simulink library "sm_humanoid_walker_lib"  (R2025b)
settings: Solver=VariableStepAuto  StartTime=0.0  StopTime=10.0  RelTol=1e-3
undefined symbols (not defined in the file or in its folder): params, X, Y, Z
libraries: sm_lib x99, nesl_utility x36, $bdroot x7, simulink x1, simulink_extras x1
(part 1 of 3)
settings Model: Creator=The MathWorks, Inc.  LastModifiedBy=jolson
settings SolverCC: AlgebraicLoopSolver=TrustRegion
settings DebuggingCC: UnconnectedInputMsg=warning  UnconnectedOutputMsg=warning  UnconnectedLineMsg=warning
settings ModelReferenceCC: EnableRefExpFcnMdlSchedulingChecks=on
settings RTWCC: GPUComputeCapability=3.5  DLArmComputeVersion=19.05

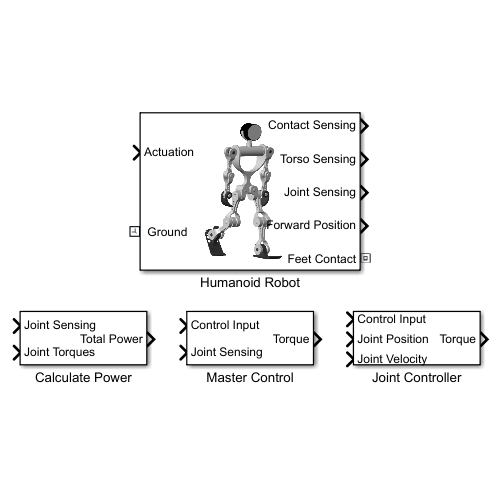
[thumbnail: Simulink's stored preview of the top-level diagram]
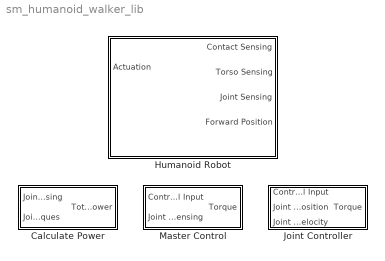
== system sm_humanoid_walker_lib ==
  Calculate Power : Subsystem
  Humanoid Robot : Subsystem  mask{contactRadius=params.contact.contactRadius, contactStiffness=params.contact.stiffness, contactDamping=params.contact.damping, contactTWidth=params.contact.transitionWidth, contactStaticFriction=params.contact.staticFriction, contactDynamicFriction=params.contact.dynamicFriction, contactCriticalVelocity=params.contact.criticalVelocity, footDensity=params.materialProperties.lowerBodyDensity, lowerLegDensity=params.materialProperties.lowerBodyDensity, upperLegDensity=params.materialProperties.lowerBodyDensity, hipDensity=params.materialProperties.lowerBodyDensity, trunkDensity=params.materialProperties.upperBodyDensity, shoulderDensity=params.materialProperties.upperBodyDensity, upperArmDensity=params.materialProperties.upperBodyDensity, lowerArmDensity=params.materialProperties.upperBodyDensity, handDensity=params.materialProperties.upperBodyDensity, headDensity=params.materialProperties.upperBodyDensity, hipUpperLimit=params.jointLimits.hipFrontalUpperLimit, hipLowerLimit=params.jointLimits.hipFrontalLowerLimit, kneeUpperLimit=params.jointLimits.kneeUpperLimit, kneeLowerLimit=params.jointLimits.kneeLowerLimit, ankleUpperLimit=params.jointLimits.ankleUpperLimit, ankleLowerLimit=params.jointLimits.ankleLowerLimit, shoulderFrontalUpperLimit=params.jointLimits.shoulderFrontalUpperLimit, shoulderFrontalLowerLimit=params.jointLimits.shoulderFrontalLowerLimit, shoulderSagittalUpperLimit=params.jointLimits.shoulderSagittalUpperLimit, shoulderSagittalLowerLimit=params.jointLimits.shoulderSagittalLowerLimit}
      mask prompts: contactRadius "Contact Sphere Radius (m)"; contactStiffness "Contact Stiffness (N/m)"; contactDamping "Contact Damping (Ns/m)"; contactTWidth "Contact Tranisiton Region Width (m)"; contactStaticFriction "Contact Static Friction"; contactDynamicFriction "Contact Dynamic Friction"; contactCriticalVelocity "Contact Critical Velocity (m/s)"; footDensity "Foot Density (kg/m^3)"; lowerLegDensity "Lower Leg Density (kg/m^3)"; upperLegDensity "Upper Leg Density (kg/m^3)"; hipDensity "Hip Density (kg/m^3)"; trunkDensity "Trunk Density (kg/m^3)"; shoulderDensity "Shoulder Density (kg/m^3)"; upperArmDensity "Upper Arm Density (kg/m^3)"; lowerArmDensity "Lower Arm Density (kg/m^3)"; handDensity "Hand Density (kg/m^3)"; headDensity "Neck / Head Density (kg/m^3)"; hipUpperLimit "Hip Frontal Upper Limit (deg)"; hipLowerLimit "Hip Frontal Lower Limit (deg)"; kneeUpperLimit "Knee Upper Limit (deg)"; kneeLowerLimit "Knee Lower Limit (deg)"; ankleUpperLimit "Ankle Upper Limit (deg)"; ankleLowerLimit "Ankle Lower Limit (deg)"; shoulderFrontalUpperLimit "Shoulder Frontal Upper Limit (deg)"; shoulderFrontalLowerLimit "Shoulder Frontal Lower Limit (deg)"; shoulderSagittalUpperLimit "Shoulder Sagittal Upper Limit (deg)"; shoulderSagittalLowerLimit "Shoulder Sagittal Lower Limit (deg)"
      mask DialogControl Container4 Prompt: Contact Parameters
      mask DialogControl Container9 Prompt: Material Properties
      mask DialogControl Container12 Prompt: Joint Parameters
      mask Display: image('sm_humanoid_robot.PNG'); % Use "Edit Image" on toolstrip to change.
  Joint Controller : Subsystem  mask{jointStiffness=0, jointDamping=0, jointUpperLimit=0, jointLowerLimit=0, jointTorqueLimit=0}
      mask prompts: jointStiffness "Joint Control Stiffness (N*m/rad)"; jointDamping "Joint Control Damping (N*m*s/rad)"; jointUpperLimit "Joint Upper Limit (deg)"; jointLowerLimit "Joint Lower Limt (deg)"; jointTorqueLimit "Joint Absolute Torque Limit (N*m)"
      mask DialogControl DescTextVar Prompt: Stiffness based joint controller.
  Master Control : Subsystem

== system sm_humanoid_walker_lib/Calculate Power ==
  Joint Sensing : Inport
  Joint Torques : Inport  Port=2
  Bus Selector1 : BusSelector  OutputSignals=signal1.signal1.rhThetaDot,signal1.signal2.rkThetaDot,signal1.signal3.raThetaDot,signal2.signal1.lhThetaDot,signal2.signal2.lkThetaDot,signal2.signal3.laThetaDot
  Mux : Mux  Inputs=6
  Product : Product
  Sum of Elements : Sum  Inputs=+
  Unit Delay : UnitDelay  SampleTime=-1  HasFrameUpgradeWarning=on
  Total Power : Outport
  wires:
  Product/1 -> Sum of Elements/1
  Joint Sensing/1 -> Bus Selector1/1
  Mux/1 -> Product/1
  Joint Torques/1 -> Product/2
  Sum of Elements/1 -> Unit Delay/1
  Bus Selector1/1 -> Mux/1  "<rhThetaDot>"
  Bus Selector1/2 -> Mux/2  "<rkThetaDot>"
  Bus Selector1/3 -> Mux/3  "<raThetaDot>"
  Bus Selector1/4 -> Mux/4  "<lhThetaDot>"
  Bus Selector1/5 -> Mux/5  "<lkThetaDot>"
  Bus Selector1/6 -> Mux/6  "<laThetaDot>"
  Unit Delay/1 -> Total Power/1

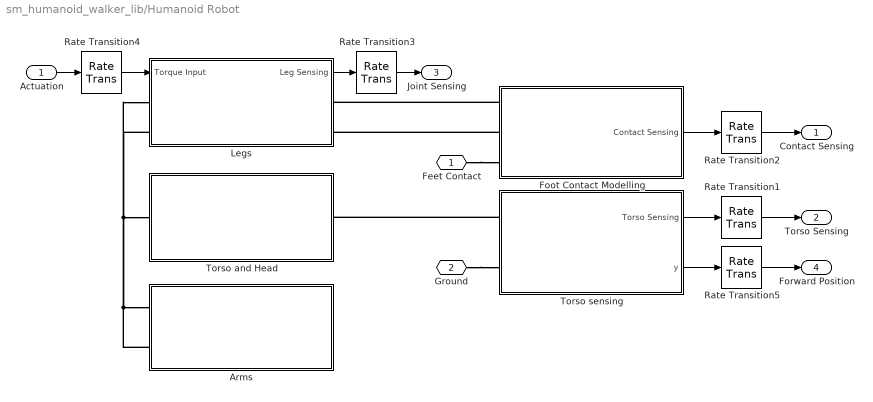
== system sm_humanoid_walker_lib/Humanoid Robot ==
  Actuation : Inport
  Arms : Subsystem
      mask Display: image('sm_humanoid_arms.PNG'); % Use "Edit Image" on toolstrip to change.
  Foot Contact Modelling : Subsystem
  Legs : Subsystem
      mask Display: image('sm_humanoid_legs.PNG'); % Use "Edit Image" on toolstrip to change.
  Rate Transition{1..5} (5 alike) : RateTransition  OutPortSampleTime=params.simulation.Ts
  Torso and Head : Subsystem
      mask Display: image('sm_humanoid_torso.PNG'); % Use "Edit Image" on toolstrip to change.
  Torso sensing : Subsystem
  Feet Contact : PMIOPort  Side=Right
  " Ground" : PMIOPort  Port=2  Side=Left
  Contact Sensing : Outport
  Torso Sensing : Outport  Port=2
  Joint Sensing : Outport  Port=3
  Forward Position : Outport  Port=4
  wires:
  Foot Contact Modelling/1(Contact Sensing) -> Rate Transition2/1
  Legs/1(Leg Sensing) -> Rate Transition3/1
  Actuation/1 -> Rate Transition4/1
  Torso sensing/1(Torso Sensing) -> Rate Transition1/1
  Rate Transition2/1 -> Contact Sensing/1
  Rate Transition1/1 -> Torso Sensing/1
  Rate Transition3/1 -> Joint Sensing/1
  Rate Transition4/1 -> Legs/1(Torque Input)
  Rate Transition5/1 -> Forward Position/1
  Torso sensing/2(y) -> Rate Transition5/1
  connections:
  Arms/LConn2 -- Legs/LConn2 -- Legs/LConn1 -- Torso and Head/LConn1 -- Arms/LConn1
  Torso sensing/LConn1 -- Torso and Head/RConn1
  Feet Contact/RConn1 -- Foot Contact Modelling/LConn3
  Foot Contact Modelling/LConn1 -- Legs/RConn1
  Foot Contact Modelling/LConn2 -- Legs/RConn2
  " Ground"/RConn1 -- Torso sensing/LConn2

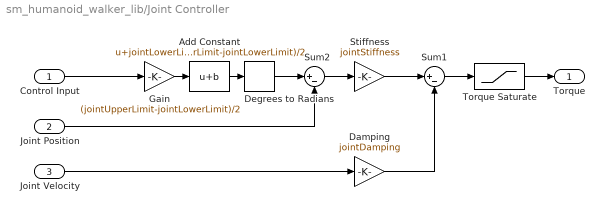
== system sm_humanoid_walker_lib/Joint Controller ==
  Control Input : Inport
  Joint Position : Inport  Port=2
  Joint Velocity : Inport  Port=3
  Add Constant : Bias  Bias=jointLowerLimit + (jointUpperLimit-jointLowerLimit)/2  SaturateOnIntegerOverflow=off
  Damping : Gain  Gain=jointDamping
  Degrees to Radians : simulink_extras/Transformations/Degrees to Radians
  Gain : Gain  Gain=(jointUpperLimit-jointLowerLimit)/2
  Stiffness : Gain  Gain=jointStiffness
  Sum1 : Sum  Inputs=|+-
  Sum2 : Sum  Inputs=|+-
  Torque Saturate : Saturate  UpperLimit=jointTorqueLimit  LowerLimit=-jointTorqueLimit  ZeroCross=off
  Torque : Outport
  wires:
  Damping/1 -> Sum1/2
  Stiffness/1 -> Sum1/1
  Add Constant/1 -> Degrees to Radians/1
  Gain/1 -> Add Constant/1
  Control Input/1 -> Gain/1
  Sum2/1 -> Stiffness/1
  Joint Velocity/1 -> Damping/1
  Sum1/1 -> Torque Saturate/1
  Torque Saturate/1 -> Torque/1
  Degrees to Radians/1 -> Sum2/1
  Joint Position/1 -> Sum2/2

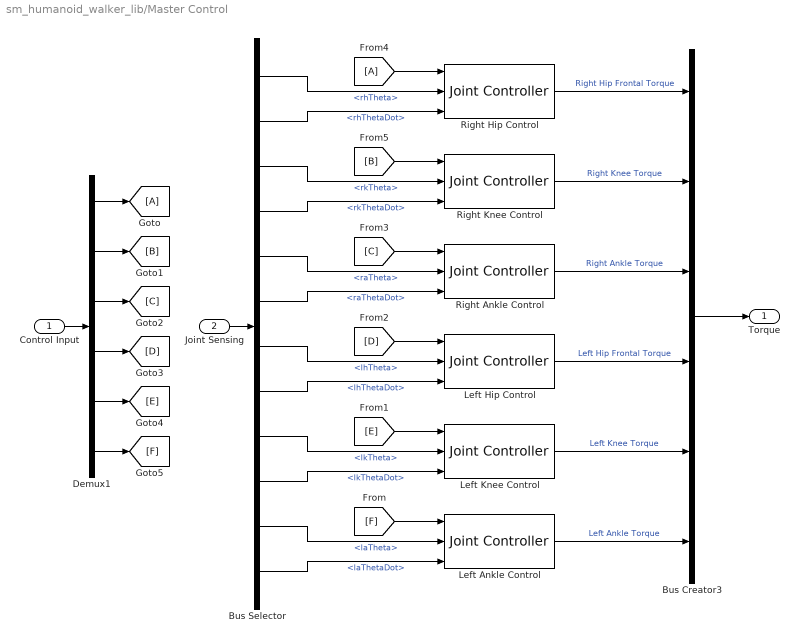
== system sm_humanoid_walker_lib/Master Control ==
  Control Input : Inport
  Joint Sensing : Inport  Port=2
  Bus Creator3 : BusCreator  Inputs=6
  Bus Selector : BusSelector  OutputSignals=signal1.signal1.rhTheta,signal1.signal1.rhThetaDot,signal1.signal2.rkTheta,signal1.signal2.rkThetaDot,signal1.signal3.raTheta,signal1.signal3.raThetaDot,signal2.signal1.lhTheta,signal2.signal1.lhThetaDot,signal2.signal2.lkTheta,signal2.signal2.lkThetaDot,signal2.signal3.laTheta,signal2.signal3.laThetaDot
  Demux1 : Demux  Outputs=6
  From4 : From
  Goto : Goto
  Left Ankle Control : $bdroot/Joint Controller  jointStiffness=params.controller.ankleStiffness  jointDamping=params.controller.ankleDamping  jointUpperLimit=params.jointLimits.ankleUpperLimit  jointLowerLimit=params.jointLimits.ankleLowerLimit  jointTorqueLimit=params.torqueLimits.ankle
  Left Hip Control : $bdroot/Joint Controller  jointStiffness=params.controller.hipFrontalStiffness  jointDamping=params.controller.hipFrontalDamping  jointUpperLimit=params.jointLimits.hipFrontalUpperLimit  jointLowerLimit=params.jointLimits.hipFrontalLowerLimit  jointTorqueLimit=params.torqueLimits.hipFrontal
  Left Knee Control : $bdroot/Joint Controller  jointStiffness=params.controller.kneeStiffness  jointDamping=params.controller.kneeDamping  jointUpperLimit=params.jointLimits.kneeUpperLimit  jointLowerLimit=params.jointLimits.kneeLowerLimit  jointTorqueLimit=params.torqueLimits.knee
  Right Ankle Control : $bdroot/Joint Controller  jointStiffness=params.controller.ankleStiffness  jointDamping=params.controller.ankleDamping  jointUpperLimit=params.jointLimits.ankleUpperLimit  jointLowerLimit=params.jointLimits.ankleLowerLimit  jointTorqueLimit=params.torqueLimits.ankle
  Right Hip Control : $bdroot/Joint Controller  jointStiffness=params.controller.hipFrontalStiffness  jointDamping=params.controller.hipFrontalDamping  jointUpperLimit=params.jointLimits.hipFrontalUpperLimit  jointLowerLimit=params.jointLimits.hipFrontalLowerLimit  jointTorqueLimit=params.torqueLimits.hipFrontal
  Right Knee Control : $bdroot/Joint Controller  jointStiffness=params.controller.kneeStiffness  jointDamping=params.controller.kneeDamping  jointUpperLimit=params.jointLimits.kneeUpperLimit  jointLowerLimit=params.jointLimits.kneeLowerLimit  jointTorqueLimit=params.torqueLimits.knee
  Torque : Outport
  wires:
  Control Input/1 -> Demux1/1
  Joint Sensing/1 -> Bus Selector/1
  Bus Creator3/1 -> Torque/1
  Bus Selector/1 -> Right Hip Control/2  "<rhTheta>"
  Bus Selector/2 -> Right Hip Control/3  "<rhThetaDot>"
  Bus Selector/3 -> Right Knee Control/2  "<rkTheta>"
  Bus Selector/4 -> Right Knee Control/3  "<rkThetaDot>"
  Bus Selector/5 -> Right Ankle Control/2  "<raTheta>"
  Bus Selector/6 -> Right Ankle Control/3  "<raThetaDot>"
  Bus Selector/7 -> Left Hip Control/2  "<lhTheta>"
  Bus Selector/8 -> Left Hip Control/3  "<lhThetaDot>"
  Bus Selector/9 -> Left Knee Control/2  "<lkTheta>"
  Bus Selector/10 -> Left Knee Control/3  "<lkThetaDot>"
  Bus Selector/11 -> Left Ankle Control/2  "<laTheta>"
  Bus Selector/12 -> Left Ankle Control/3  "<laThetaDot>"
  Right Ankle Control/1 -> Bus Creator3/3  "Right Ankle Torque"
  Right Knee Control/1 -> Bus Creator3/2  "Right Knee Torque"
  Right Hip Control/1 -> Bus Creator3/1  "Right Hip Frontal Torque"
  Left Knee Control/1 -> Bus Creator3/5  "Left Knee Torque"
  Left Hip Control/1 -> Bus Creator3/4  "Left Hip Frontal Torque"
  Left Ankle Control/1 -> Bus Creator3/6  "Left Ankle Torque"
  Demux1/1 -> Goto/1
  Demux1/6 -> [F]
  Demux1/5 -> [E]
  Demux1/4 -> [D]
  Demux1/3 -> [C]
  Demux1/2 -> [B]
  [F] -> Left Ankle Control/1
  [E] -> Left Knee Control/1
  [D] -> Left Hip Control/1
  [C] -> Right Ankle Control/1
  From4/1 -> Right Hip Control/1
  [B] -> Right Knee Control/1

== system sm_humanoid_walker_lib/Humanoid Robot/Arms ==
  Left Arm : Subsystem
  Right Arm : Subsystem
  Right Shoulder : PMIOPort  Side=Left
  Left Shoulder : PMIOPort  Port=2  Side=Left
  connections:
  Right Arm/LConn1 -- Right Shoulder/RConn1
  Left Arm/LConn1 -- Left Shoulder/RConn1

== system sm_humanoid_walker_lib/Humanoid Robot/Foot Contact Modelling ==
  Bus Creator : BusCreator  Inputs=2
  Left Foot Contact : $bdroot/Humanoid Robot/Foot Contact Modelling/Right Foot Contact  SystemSampleTime=-1  VariantActivationTime=update diagram  EmptyChoice=off  PassThrough=off  PassThroughVariantControl=(default)  EmptyChoiceVariantControl=(default)  AllowFlexibleInterface=on  Latency=0  AutoFrameSizeCalculation=off
  Right Foot Contact : Subsystem
  Right Foot Contact Points : PMIOPort  Side=Left
  Left Foot Contact Points : PMIOPort  Port=2  Side=Left
  Feet Contact : PMIOPort  Port=3  Side=Left
  Contact Sensing : Outport
  wires:
  Left Foot Contact/1 -> Bus Creator/2  "leftContact"
  Right Foot Contact/1(Foot Force) -> Bus Creator/1  "rightContact"
  Bus Creator/1 -> Contact Sensing/1
  connections:
  Right Foot Contact/LConn1 -- Right Foot Contact Points/RConn1
  Right Foot Contact/RConn1 -- Left Foot Contact/RConn1 -- Feet Contact/RConn1
  Left Foot Contact/LConn1 -- Left Foot Contact Points/RConn1

== system sm_humanoid_walker_lib/Humanoid Robot/Legs ==
  Torque Input : Inport
  Bus Creator1 : BusCreator  Inputs=2
  Demux : Demux  Outputs=2
  Left Leg : Subsystem
  Right leg : Subsystem
  Right Hip : PMIOPort  Side=Left
  Right Foot : PMIOPort  Port=2  Side=Right
  Left Foot : PMIOPort  Port=3  Side=Right
  Left Hip : PMIOPort  Port=4  Side=Left
  Leg Sensing : Outport
  wires:
  Demux/1 -> Right leg/1(Torque Input)
  Torque Input/1 -> Demux/1
  Left Leg/1(Sensing) -> Bus Creator1/2
  Right leg/1(Sensing) -> Bus Creator1/1
  Bus Creator1/1 -> Leg Sensing/1
  Demux/2 -> Left Leg/1(Torque Input)
  connections:
  Left Hip/RConn1 -- Left Leg/LConn1
  Right Foot/RConn1 -- Right leg/RConn1
  Left Foot/RConn1 -- Left Leg/RConn1
  Right Hip/RConn1 -- Right leg/LConn1

== system sm_humanoid_walker_lib/Humanoid Robot/Torso and Head ==
  Cover : sm_lib/Body Elements/File Solid  ExtGeomFileName=sm_humanoid_walker_cover.stp  UnitType=FromFile  ExtGeomFileUnits=m  StepReaderType=HEX  ExportConvexHullGeometry=off  InertiaType=CalculateFromGeometry  BasedOnType=Density  Density=headDensity  DensityUnits=kg/m^3  Mass=0  MassUnits=kg  CenterOfMass=[0, 0, 0]  CenterOfMassUnits=m  MomentsOfInertia=[0, 0, 0]  MomentsOfInertiaUnits=kg*m^2  ProductsOfInertia=[0, 0, 0]  ProductsOfInertiaUnits=kg*m^2  GraphicType=FromGeometry  MarkerShape=Sphere  MarkerSize=10  GraphicVisPropType=SimpleVisualProperties  GraphicDiffuseColor=[1, 1, 1]  GraphicOpacity=1  GraphicSpecularColor=[0.5 0.5 0.5 1.0]  GraphicAmbientColor=[0.15 0.15 0.15 1.0]  GraphicEmissiveColor=[0.0 0.0 0.0 1.0]  GraphicShininess=75  DoExposeReferenceFrame=on  SerializedFrames=<Frames/>
  Head : sm_lib/Body Elements/File Solid  ExtGeomFileName=sm_humanoid_walker_head.stp  UnitType=FromFile  ExtGeomFileUnits=m  StepReaderType=HEX  ExportConvexHullGeometry=off  InertiaType=CalculateFromGeometry  BasedOnType=Density  Density=headDensity  DensityUnits=kg/m^3  Mass=0  MassUnits=kg  CenterOfMass=[0, 0, 0]  CenterOfMassUnits=m  MomentsOfInertia=[0, 0, 0]  MomentsOfInertiaUnits=kg*m^2  ProductsOfInertia=[0, 0, 0]  ProductsOfInertiaUnits=kg*m^2  GraphicType=FromGeometry  MarkerShape=Sphere  MarkerSize=10  GraphicVisPropType=SimpleVisualProperties  GraphicDiffuseColor=[0.0 0.0 0.0]  GraphicOpacity=1  GraphicSpecularColor=[0.5 0.5 0.5 1.0]  GraphicAmbientColor=[0.15 0.15 0.15 1.0]  GraphicEmissiveColor=[0.0 0.0 0.0 1.0]  GraphicShininess=75  DoExposeReferenceFrame=on  SerializedFrames=<Frames/>
  Head Origin Transformation : sm_lib/Frames and Transforms/Rigid Transform  RotationMethod=RotationSequence  FollAlignAxisA=+X  BaseAlignAxisA=+Y  FollAlignAxisB=+Y  BaseAlignAxisB=+Z  RotationStandardAxis=+Z  RotationAngle=0.0  RotationAngleUnits=deg  RotationArbitraryAxis=[0 0 1]  RotationSequenceAxes=BaseAxes  RotationSequence=XYZ  RotationSequenceAngles=[0, 0, 0]  RotationSequenceAnglesUnits=rad  RotationMatrix=[1 0 0; 0 1 0; 0 0 1]  Quaternion=[1 0 0 0]  TranslationMethod=Cartesian  TranslationCartesianOffset=[0, 0, 0.06414]*3.5  TranslationCartesianOffsetUnits=m  TranslationStandardAxis=+Z  TranslationStandardOffset=0  TranslationStandardOffsetUnits=m  TranslationROffset=0  TranslationROffsetUnits=m  TranslationThetaOffset=0  TranslationThetaOffsetUnits=deg  TranslationZOffset=0  TranslationZOffsetUnits=m
  Neck : sm_lib/Body Elements/File Solid  ExtGeomFileName=sm_humanoid_walker_neck.stp  UnitType=FromFile  ExtGeomFileUnits=m  StepReaderType=HEX  ExportConvexHullGeometry=off  InertiaType=CalculateFromGeometry  BasedOnType=Density  Density=headDensity  DensityUnits=kg/m^3  Mass=0  MassUnits=kg  CenterOfMass=[0, 0, 0]  CenterOfMassUnits=m  MomentsOfInertia=[0, 0, 0]  MomentsOfInertiaUnits=kg*m^2  ProductsOfInertia=[0, 0, 0]  ProductsOfInertiaUnits=kg*m^2  GraphicType=FromGeometry  MarkerShape=Sphere  MarkerSize=10  GraphicVisPropType=SimpleVisualProperties  GraphicDiffuseColor=[0.0 0.0 0.0]  GraphicOpacity=1  GraphicSpecularColor=[0.5 0.5 0.5 1.0]  GraphicAmbientColor=[0.15 0.15 0.15 1.0]  GraphicEmissiveColor=[0.0 0.0 0.0 1.0]  GraphicShininess=75  DoExposeReferenceFrame=on  SerializedFrames=<Frames/>
  Neck Origin Tranformation : sm_lib/Frames and Transforms/Rigid Transform  RotationMethod=RotationSequence  FollAlignAxisA=+X  BaseAlignAxisA=+Y  FollAlignAxisB=+Y  BaseAlignAxisB=+Z  RotationStandardAxis=+Z  RotationAngle=0.0  RotationAngleUnits=deg  RotationArbitraryAxis=[0 0 1]  RotationSequenceAxes=BaseAxes  RotationSequence=XYZ  RotationSequenceAngles=[0, 0, 0]  RotationSequenceAnglesUnits=rad  RotationMatrix=[1 0 0; 0 1 0; 0 0 1]  Quaternion=[1 0 0 0]  TranslationMethod=Cartesian  TranslationCartesianOffset=[0, 0, 0.01016]*3.5  TranslationCartesianOffsetUnits=m  TranslationStandardAxis=+Z  TranslationStandardOffset=0  TranslationStandardOffsetUnits=m  TranslationROffset=0  TranslationROffsetUnits=m  TranslationThetaOffset=0  TranslationThetaOffsetUnits=deg  TranslationZOffset=0  TranslationZOffsetUnits=m
  Shoulder : sm_lib/Body Elements/File Solid  ExtGeomFileName=sm_humanoid_walker_shoulder.stp  UnitType=FromFile  ExtGeomFileUnits=m  StepReaderType=HEX  ExportConvexHullGeometry=off  InertiaType=CalculateFromGeometry  BasedOnType=Density  Density=shoulderDensity  DensityUnits=kg/m^3  Mass=0  MassUnits=kg  CenterOfMass=[0, 0, 0]  CenterOfMassUnits=m  MomentsOfInertia=[0, 0, 0]  MomentsOfInertiaUnits=kg*m^2  ProductsOfInertia=[0, 0, 0]  ProductsOfInertiaUnits=kg*m^2  GraphicType=FromGeometry  MarkerShape=Sphere  MarkerSize=10  GraphicVisPropType=SimpleVisualProperties  GraphicDiffuseColor=[1.0 0.6 0.6]  GraphicOpacity=1  GraphicSpecularColor=[0.5 0.5 0.5 1.0]  GraphicAmbientColor=[0.15 0.15 0.15 1.0]  GraphicEmissiveColor=[0.0 0.0 0.0 1.0]  GraphicShininess=75  DoExposeReferenceFrame=on  SerializedFrames=<Frames/>
  Shoulder Origin Transformation : sm_lib/Frames and Transforms/Rigid Transform  RotationMethod=RotationSequence  FollAlignAxisA=+X  BaseAlignAxisA=+Y  FollAlignAxisB=+Y  BaseAlignAxisB=+Z  RotationStandardAxis=+Z  RotationAngle=0.0  RotationAngleUnits=deg  RotationArbitraryAxis=[0 0 1]  RotationSequenceAxes=BaseAxes  RotationSequence=XYZ  RotationSequenceAngles=[0, 0, 0]  RotationSequenceAnglesUnits=rad  RotationMatrix=[1 0 0; 0 1 0; 0 0 1]  Quaternion=[1 0 0 0]  TranslationMethod=Cartesian  TranslationCartesianOffset=[0, 0, -0.0399]*3.5  TranslationCartesianOffsetUnits=m  TranslationStandardAxis=+Z  TranslationStandardOffset=0  TranslationStandardOffsetUnits=m  TranslationROffset=0  TranslationROffsetUnits=m  TranslationThetaOffset=0  TranslationThetaOffsetUnits=deg  TranslationZOffset=0  TranslationZOffsetUnits=m
  Trunk : sm_lib/Body Elements/File Solid  ExtGeomFileName=sm_humanoid_walker_trunk.stp  UnitType=FromFile  ExtGeomFileUnits=km  StepReaderType=HEX  ExportConvexHullGeometry=off  InertiaType=CalculateFromGeometry  BasedOnType=Density  Density=trunkDensity  DensityUnits=kg/m^3  Mass=0  MassUnits=kg  CenterOfMass=[0, 0, 0]  CenterOfMassUnits=m  MomentsOfInertia=[0, 0, 0]  MomentsOfInertiaUnits=kg*m^2  ProductsOfInertia=[0, 0, 0]  ProductsOfInertiaUnits=kg*m^2  GraphicType=FromGeometry  MarkerShape=Sphere  MarkerSize=10  GraphicVisPropType=SimpleVisualProperties  GraphicDiffuseColor=[1.0 0.2 0.2]  GraphicOpacity=1  GraphicSpecularColor=[0.5 0.5 0.5 1.0]  GraphicAmbientColor=[0.15 0.15 0.15 1.0]  GraphicEmissiveColor=[0.0 0.0 0.0 1.0]  GraphicShininess=75  DoExposeReferenceFrame=on  SerializedFrames=<Frames/>
  Torso : PMIOPort  Side=Left
  Torso Ref : PMIOPort  Port=2  Side=Right
  connections:
  Shoulder Origin Transformation/LConn1 -- Torso Ref/RConn1 -- Torso/RConn1 -- Trunk/RConn1
  Head/RConn1 -- Head Origin Transformation/RConn1 -- Cover/RConn1
  Shoulder/RConn1 -- Shoulder Origin Transformation/RConn1 -- Neck Origin Tranformation/LConn1
  Neck Origin Tranformation/RConn1 -- Head Origin Transformation/LConn1 -- Neck/RConn1

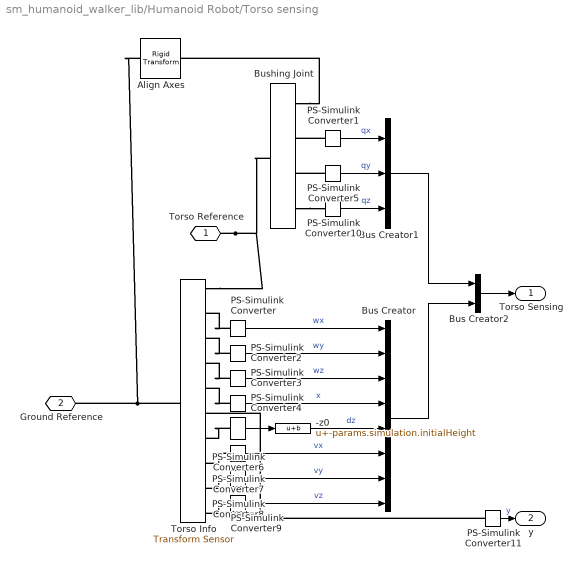
== system sm_humanoid_walker_lib/Humanoid Robot/Torso sensing ==
  -z0 : Bias  Bias=-params.simulation.initialHeight  SaturateOnIntegerOverflow=off
  Align Axes : sm_lib/Frames and Transforms/Rigid Transform  RotationMethod=StandardAxis  FollAlignAxisA=+X  BaseAlignAxisA=+Y  FollAlignAxisB=+Y  BaseAlignAxisB=+Z  RotationStandardAxis=+Z  RotationAngle=180  RotationAngleUnits=deg  RotationArbitraryAxis=[0 0 1]  RotationSequenceAxes=FollowerAxes  RotationSequence=XYX  RotationSequenceAngles=[0 0 0]  RotationSequenceAnglesUnits=deg  RotationMatrix=[1 0 0; 0 1 0; 0 0 1]  Quaternion=[1 0 0 0]  TranslationMethod=None  TranslationCartesianOffset=[0 0 0]  TranslationCartesianOffsetUnits=m  TranslationStandardAxis=+Z  TranslationStandardOffset=0  TranslationStandardOffsetUnits=m  TranslationROffset=0  TranslationROffsetUnits=m  TranslationThetaOffset=0  TranslationThetaOffsetUnits=deg  TranslationZOffset=0  TranslationZOffsetUnits=m
  Bus Creator : BusCreator  Inputs=8
  Bus Creator1 : BusCreator  Inputs=3
  Bus Creator2 : BusCreator  Inputs=2
  Bushing Joint : sm_lib/Joints/Bushing Joint  JointMode=Normal  CompositeWrenchDir=FollowerOnBase  CompositeWrenchFrame=BaseFrame  SenseConstraintForce=off  SenseConstraintTorque=off  SenseTotalForce=off  SenseTotalTorque=off  PxPositionTargetSpecify=off  PxPositionTargetPriority=High  PxPositionTargetValue=0  PxPositionTargetValueUnits=m  PxVelocityTargetSpecify=off  PxVelocityTargetPriority=High  PxVelocityTargetValue=0  PxVelocityTargetValueUnits=m/s  PxEquilibriumPosition=0  PxEquilibriumPositionUnits=m  PxSpringStiffness=0  PxSpringStiffnessUnits=N/m  PxDampingCoefficient=0  PxDampingCoefficientUnits=N/(m/s)  PxLowerLimitSpecify=off  PxLowerLimitBound=-0.02  PxLowerLimitBoundUnits=m  PxLowerLimitStiffness=1e6  PxLowerLimitStiffnessUnits=N/m  PxLowerLimitDamping=1e3  PxLowerLimitDampingUnits=N/(m/s)  PxLowerLimitTransitionRegionWidth=1e-4  PxLowerLimitTransitionRegionWidthUnits=m  PxUpperLimitSpecify=off  PxUpperLimitBound=0.02  PxUpperLimitBoundUnits=m  PxUpperLimitStiffness=1e6  PxUpperLimitStiffnessUnits=N/m  PxUpperLimitDamping=1e3  PxUpperLimitDampingUnits=N/(m/s)  PxUpperLimitTransitionRegionWidth=1e-4  PxUpperLimitTransitionRegionWidthUnits=m  PxTorqueActuationMode=NoTorque  PxMotionActuationMode=ComputedMotion  PxSensePosition=off  PxSenseVelocity=off  PxSenseAcceleration=off  PxSenseTorqueForce=off  PxSenseLowerLimitTorqueForce=off  PxSenseUpperLimitTorqueForce=off  PyPositionTargetSpecify=off  PyPositionTargetPriority=High  PyPositionTargetValue=0  PyPositionTargetValueUnits=m  PyVelocityTargetSpecify=off  PyVelocityTargetPriority=High  PyVelocityTargetValue=0  PyVelocityTargetValueUnits=m/s  PyEquilibriumPosition=0  PyEquilibriumPositionUnits=m  PySpringStiffness=0  PySpringStiffnessUnits=N/m  PyDampingCoefficient=0  PyDampingCoefficientUnits=N/(m/s)  PyLowerLimitSpecify=off  PyLowerLimitBound=-1  PyLowerLimitBoundUnits=m  PyLowerLimitStiffness=1e6  PyLowerLimitStiffnessUnits=N/m  PyLowerLimitDamping=1e3  PyLowerLimitDampingUnits=N/(m/s)  PyLowerLimitTransitionRegionWidth=1e-4  PyLowerLimitTransitionRegionWidthUnits=m  PyUpperLimitSpecify=off  PyUpperLimitBound=1  PyUpperLimitBoundUnits=m  PyUpperLimitStiffness=1e6  PyUpperLimitStiffnessUnits=N/m  PyUpperLimitDamping=1e3  PyUpperLimitDampingUnits=N/(m/s)  PyUpperLimitTransitionRegionWidth=1e-4  PyUpperLimitTransitionRegionWidthUnits=m  PyTorqueActuationMode=NoTorque  PyMotionActuationMode=ComputedMotion  PySensePosition=off  PySenseVelocity=off  PySenseAcceleration=off  PySenseTorqueForce=off  PySenseLowerLimitTorqueForce=off  PySenseUpperLimitTorqueForce=off  PzPositionTargetSpecify=on  PzPositionTargetPriority=High  PzPositionTargetValue=-params.simulation.initialHeight  PzPositionTargetValueUnits=m  PzVelocityTargetSpecify=off  PzVelocityTargetPriority=High  PzVelocityTargetValue=0  PzVelocityTargetValueUnits=m/s  PzEquilibriumPosition=0  PzEquilibriumPositionUnits=m  PzSpringStiffness=0  PzSpringStiffnessUnits=N/m  PzDampingCoefficient=params.simulation.worldDamping  PzDampingCoefficientUnits=N/(m/s)  PzLowerLimitSpecify=off  PzLowerLimitBound=-1  PzLowerLimitBoundUnits=m  PzLowerLimitStiffness=1e6  PzLowerLimitStiffnessUnits=N/m  PzLowerLimitDamping=1e3  PzLowerLimitDampingUnits=N/(m/s)  PzLowerLimitTransitionRegionWidth=1e-4  PzLowerLimitTransitionRegionWidthUnits=m  PzUpperLimitSpecify=off  PzUpperLimitBound=1  PzUpperLimitBoundUnits=m  PzUpperLimitStiffness=1e6  PzUpperLimitStiffnessUnits=N/m  PzUpperLimitDamping=1e3  PzUpperLimitDampingUnits=N/(m/s)  PzUpperLimitTransitionRegionWidth=1e-4  PzUpperLimitTransitionRegionWidthUnits=m  PzTorqueActuationMode=NoTorque  PzMotionActuationMode=ComputedMotion  PzSensePosition=off  PzSenseVelocity=off  PzSenseAcceleration=off  PzSenseTorqueForce=off  PzSenseLowerLimitTorqueForce=off  PzSenseUpperLimitTorqueForce=off  RxPositionTargetSpecify=on  RxPositionTargetPriority=High  RxPositionTargetValue=-10  RxPositionTargetValueUnits=deg  RxVelocityTargetSpecify=off  RxVelocityTargetPriority=High  RxVelocityTargetValue=0  RxVelocityTargetValueUnits=deg/s  RxEquilibriumPosition=0  RxEquilibriumPositionUnits=deg  RxSpringStiffness=0  RxSpringStiffnessUnits=N*m/deg  RxDampingCoefficient=params.simulation.worldDamping  RxDampingCoefficientUnits=N*m/(deg/s)  RxLowerLimitSpecify=off  RxLowerLimitBound=-90  RxLowerLimitBoundUnits=deg  RxLowerLimitStiffness=1e4  RxLowerLimitStiffnessUnits=N*m/deg  RxLowerLimitDamping=10  RxLowerLimitDampingUnits=N*m/(deg/s)  RxLowerLimitTransitionRegionWidth=0.1  RxLowerLimitTransitionRegionWidthUnits=deg  RxUpperLimitSpecify=off  RxUpperLimitBound=90  RxUpperLimitBoundUnits=deg  RxUpperLimitStiffness=1e4  RxUpperLimitStiffnessUnits=N*m/deg  RxUpperLimitDamping=10  RxUpperLimitDampingUnits=N*m/(deg/s)  RxUpperLimitTransitionRegionWidth=0.1  RxUpperLimitTransitionRegionWidthUnits=deg  RxTorqueActuationMode=NoTorque  RxMotionActuationMode=ComputedMotion  RxSensePosition=on  RxSenseVelocity=off  RxSenseAcceleration=off  RxSenseTorqueForce=off  RxSenseLowerLimitTorqueForce=off  RxSenseUpperLimitTorqueForce=off  RyPositionTargetSpecify=off  RyPositionTargetPriority=High  RyPositionTargetValue=0  RyPositionTargetValueUnits=deg  RyVelocityTargetSpecify=off  RyVelocityTargetPriority=High  RyVelocityTargetValue=0  RyVelocityTargetValueUnits=deg/s  RyEquilibriumPosition=0  RyEquilibriumPositionUnits=deg  RySpringStiffness=0  RySpringStiffnessUnits=N*m/deg  RyDampingCoefficient=params.simulation.worldDamping  RyDampingCoefficientUnits=N*m/(deg/s)  RyLowerLimitSpecify=off  RyLowerLimitBound=-90  RyLowerLimitBoundUnits=deg  RyLowerLimitStiffness=1e4  RyLowerLimitStiffnessUnits=N*m/deg  RyLowerLimitDamping=10  RyLowerLimitDampingUnits=N*m/(deg/s)  RyLowerLimitTransitionRegionWidth=0.1  RyLowerLimitTransitionRegionWidthUnits=deg  RyUpperLimitSpecify=off  RyUpperLimitBound=90  RyUpperLimitBoundUnits=deg  RyUpperLimitStiffness=1e4  RyUpperLimitStiffnessUnits=N*m/deg  RyUpperLimitDamping=10  RyUpperLimitDampingUnits=N*m/(deg/s)  RyUpperLimitTransitionRegionWidth=0.1  RyUpperLimitTransitionRegionWidthUnits=deg  RyTorqueActuationMode=NoTorque  RyMotionActuationMode=ComputedMotion  RySensePosition=on  RySenseVelocity=off  RySenseAcceleration=off  RySenseTorqueForce=off  RySenseLowerLimitTorqueForce=off  RySenseUpperLimitTorqueForce=off  RzPositionTargetSpecify=on  RzPositionTargetPriority=High  RzPositionTargetValue=0  RzPositionTargetValueUnits=deg  RzVelocityTargetSpecify=off  RzVelocityTargetPriority=High  RzVelocityTargetValue=0  RzVelocityTargetValueUnits=deg/s  RzEquilibriumPosition=0  RzEquilibriumPositionUnits=deg  RzSpringStiffness=0  RzSpringStiffnessUnits=N*m/deg  RzDampingCoefficient=params.simulation.worldDamping  RzDampingCoefficientUnits=N*m/(deg/s)  RzLowerLimitSpecify=off  RzLowerLimitBound=-90  RzLowerLimitBoundUnits=deg  RzLowerLimitStiffness=1e4  RzLowerLimitStiffnessUnits=N*m/deg  RzLowerLimitDamping=10  RzLowerLimitDampingUnits=N*m/(deg/s)  RzLowerLimitTransitionRegionWidth=0.1  RzLowerLimitTransitionRegionWidthUnits=deg  RzUpperLimitSpecify=off  RzUpperLimitBound=90  RzUpperLimitBoundUnits=deg  RzUpperLimitStiffness=1e4  RzUpperLimitStiffnessUnits=N*m/deg  RzUpperLimitDamping=10  RzUpperLimitDampingUnits=N*m/(deg/s)  RzUpperLimitTransitionRegionWidth=0.1  RzUpperLimitTransitionRegionWidthUnits=deg  RzTorqueActuationMode=NoTorque  RzMotionActuationMode=ComputedMotion  RzSensePosition=on  RzSenseVelocity=off  RzSenseAcceleration=off  RzSenseTorqueForce=off  RzSenseLowerLimitTorqueForce=off  RzSenseUpperLimitTorqueForce=off
  PS-Simulink Converter{,1..11} (12 alike) : nesl_utility/PS-Simulink Converter  PhysicalDomain=network_engine_domain  SubClassName=ps_output  LeftPortType=input  RightPortType=output  PseudoPeriodic=off  Frequencies=[]  VectorFormat=1-D array  Unit=inherit  AffineConversion=off
  Torso Info : sm_lib/Frames and Transforms/Transform Sensor  MeasurementFrame=World  RotationSequence=XYX  SenseAngle=off  SenseAxis=off  SenseQ=off  SenseR=off  SenseRotationSequence=off  SenseOmegaX=on  SenseOmegaY=on  SenseOmegaZ=on  SenseOmega=off  SenseQDot=off  SenseRDot=off  SenseRotationSequenceDot=off  SenseAlphaX=off  SenseAlphaY=off  SenseAlphaZ=off  SenseAlpha=off  SenseQDDot=off  SenseRDDot=off  SenseX=on  SenseY=on  SenseZ=on  SenseXYZ=off  SenseRad=off  SenseAzim=off  SenseDist=off  SenseInc=off  SenseXDot=on  SenseYDot=on  SenseZDot=on  SenseXYZDot=off  SenseRadDot=off  SenseAzimDot=off  SenseDistDot=off  SenseIncDot=off  SenseXDDot=off  SenseYDDot=off  SenseZDDot=off  SenseXYZDDot=off  SenseRadDDot=off  SenseAzimDDot=off  SenseDistDDot=off  SenseIncDDot=off
  Torso Reference : PMIOPort  Side=Left
  Ground Reference : PMIOPort  Port=2  Side=Left
  Torso Sensing : Outport
  y : Outport  Port=2
  wires:
  Bus Creator/1 -> Bus Creator2/2
  Bus Creator2/1 -> Torso Sensing/1
  PS-Simulink Converter1/1 -> Bus Creator1/1  "qx"
  PS-Simulink Converter5/1 -> Bus Creator1/2  "qy"
  Bus Creator1/1 -> Bus Creator2/1
  PS-Simulink Converter10/1 -> Bus Creator1/3  "qz"
  -z0/1 -> Bus Creator/5  "dz"
  PS-Simulink Converter9/1 -> Bus Creator/8  "vz"
  PS-Simulink Converter8/1 -> Bus Creator/7  "vy"
  PS-Simulink Converter7/1 -> Bus Creator/6  "vx"
  PS-Simulink Converter6/1 -> -z0/1
  PS-Simulink Converter4/1 -> Bus Creator/4  "x"
  PS-Simulink Converter3/1 -> Bus Creator/3  "wz"
  PS-Simulink Converter2/1 -> Bus Creator/2  "wy"
  PS-Simulink Converter/1 -> Bus Creator/1  "wx"
  PS-Simulink Converter11/1 -> y/1  "y"
  connections:
  Torso Info/LConn1 -- Ground Reference/RConn1 -- Align Axes/LConn1
  PS-Simulink Converter1/LConn1 -- Bushing Joint/RConn2
  PS-Simulink Converter5/LConn1 -- Bushing Joint/RConn3
  Bushing Joint/RConn4 -- PS-Simulink Converter10/LConn1
  PS-Simulink Converter2/LConn1 -- Torso Info/RConn3
  PS-Simulink Converter3/LConn1 -- Torso Info/RConn4
  PS-Simulink Converter4/LConn1 -- Torso Info/RConn5
  PS-Simulink Converter/LConn1 -- Torso Info/RConn2
  Bushing Joint/RConn1 -- Align Axes/RConn1
  Torso Reference/RConn1 -- Bushing Joint/LConn1 -- Torso Info/RConn1
  PS-Simulink Converter9/LConn1 -- Torso Info/RConn10
  PS-Simulink Converter8/LConn1 -- Torso Info/RConn9
  PS-Simulink Converter7/LConn1 -- Torso Info/RConn8
  PS-Simulink Converter6/LConn1 -- Torso Info/RConn7
  PS-Simulink Converter11/LConn1 -- Torso Info/RConn6

== system sm_humanoid_walker_lib/Humanoid Robot/Arms/Left Arm ==
  Elbow Joint : Subsystem
  Hand : sm_lib/Body Elements/File Solid  ExtGeomFileName=sm_humanoid_walker_hand.stp  UnitType=FromFile  ExtGeomFileUnits=m  StepReaderType=HEX  ExportConvexHullGeometry=off  InertiaType=CalculateFromGeometry  BasedOnType=Density  Density=handDensity  DensityUnits=kg/m^3  Mass=0  MassUnits=kg  CenterOfMass=[0, 0, 0]  CenterOfMassUnits=m  MomentsOfInertia=[0, 0, 0]  MomentsOfInertiaUnits=kg*m^2  ProductsOfInertia=[0, 0, 0]  ProductsOfInertiaUnits=kg*m^2  GraphicType=FromGeometry  MarkerShape=Sphere  MarkerSize=10  GraphicVisPropType=SimpleVisualProperties  GraphicDiffuseColor=[0.3, 0.3, 0.3]  GraphicOpacity=1  GraphicSpecularColor=[0.5 0.5 0.5 1.0]  GraphicAmbientColor=[0.15 0.15 0.15 1.0]  GraphicEmissiveColor=[0.0 0.0 0.0 1.0]  GraphicShininess=75  DoExposeReferenceFrame=on  SerializedFrames=<Frames/>
  Lower Arm : sm_lib/Body Elements/File Solid  ExtGeomFileName=sm_humanoid_walker_lower_arm.stp  UnitType=FromFile  ExtGeomFileUnits=m  StepReaderType=HEX  ExportConvexHullGeometry=off  InertiaType=CalculateFromGeometry  BasedOnType=Density  Density=lowerArmDensity  DensityUnits=kg/m^3  Mass=0  MassUnits=kg  CenterOfMass=[0, 0, 0]  CenterOfMassUnits=m  MomentsOfInertia=[0, 0, 0]  MomentsOfInertiaUnits=kg*m^2  ProductsOfInertia=[0, 0, 0]  ProductsOfInertiaUnits=kg*m^2  GraphicType=FromGeometry  MarkerShape=Sphere  MarkerSize=10  GraphicVisPropType=SimpleVisualProperties  GraphicDiffuseColor=[1, 1, 1]  GraphicOpacity=1  GraphicSpecularColor=[0.5 0.5 0.5 1.0]  GraphicAmbientColor=[0.15 0.15 0.15 1.0]  GraphicEmissiveColor=[0.0 0.0 0.0 1.0]  GraphicShininess=75  DoExposeReferenceFrame=on  SerializedFrames=<Frames/>
  Shoulder Frontal Joint : Subsystem
  Shoulder Sagittal Joint : Subsystem
  Shoulder Swivel : sm_lib/Body Elements/File Solid  ExtGeomFileName=sm_humanoid_walker_shoulder_swivel.stp  UnitType=FromFile  ExtGeomFileUnits=m  StepReaderType=HEX  ExportConvexHullGeometry=off  InertiaType=CalculateFromGeometry  BasedOnType=Density  Density=shoulderDensity  DensityUnits=kg/m^3  Mass=0  MassUnits=kg  CenterOfMass=[0, 0, 0]  CenterOfMassUnits=m  MomentsOfInertia=[0, 0, 0]  MomentsOfInertiaUnits=kg*m^2  ProductsOfInertia=[0, 0, 0]  ProductsOfInertiaUnits=kg*m^2  GraphicType=FromGeometry  MarkerShape=Sphere  MarkerSize=10  GraphicVisPropType=SimpleVisualProperties  GraphicDiffuseColor=[0.3, 0.3, 0.3]  GraphicOpacity=1  GraphicSpecularColor=[0.5 0.5 0.5 1.0]  GraphicAmbientColor=[0.15 0.15 0.15 1.0]  GraphicEmissiveColor=[0.0 0.0 0.0 1.0]  GraphicShininess=75  DoExposeReferenceFrame=on  SerializedFrames=<Frames/>
  Upper Arm : sm_lib/Body Elements/File Solid  ExtGeomFileName=sm_humanoid_walker_upper_arm.stp  UnitType=FromFile  ExtGeomFileUnits=m  StepReaderType=HEX  ExportConvexHullGeometry=off  InertiaType=CalculateFromGeometry  BasedOnType=Density  Density=upperArmDensity  DensityUnits=kg/m^3  Mass=0  MassUnits=kg  CenterOfMass=[0, 0, 0]  CenterOfMassUnits=m  MomentsOfInertia=[0, 0, 0]  MomentsOfInertiaUnits=kg*m^2  ProductsOfInertia=[0, 0, 0]  ProductsOfInertiaUnits=kg*m^2  GraphicType=FromGeometry  MarkerShape=Sphere  MarkerSize=10  GraphicVisPropType=SimpleVisualProperties  GraphicDiffuseColor=[1, 1, 1]  GraphicOpacity=1  GraphicSpecularColor=[0.5 0.5 0.5 1.0]  GraphicAmbientColor=[0.15 0.15 0.15 1.0]  GraphicEmissiveColor=[0.0 0.0 0.0 1.0]  GraphicShininess=75  DoExposeReferenceFrame=on  SerializedFrames=<Frames/>
  Wrist Joint : Subsystem
  Left Shoulder : PMIOPort  Side=Left
  connections:
  Shoulder Sagittal Joint/RConn1 -- Upper Arm/RConn1 -- Elbow Joint/LConn1
  Shoulder Frontal Joint/RConn1 -- Shoulder Swivel/RConn1 -- Shoulder Sagittal Joint/LConn1
  Shoulder Frontal Joint/LConn1 -- Left Shoulder/RConn1
  Elbow Joint/RConn1 -- Lower Arm/RConn1 -- Wrist Joint/LConn1
  Hand/RConn1 -- Wrist Joint/RConn1

== system sm_humanoid_walker_lib/Humanoid Robot/Arms/Right Arm ==
  Elbow Joint : Subsystem
  Hand : sm_lib/Body Elements/File Solid  ExtGeomFileName=sm_humanoid_walker_hand.stp  UnitType=FromFile  ExtGeomFileUnits=m  StepReaderType=HEX  ExportConvexHullGeometry=off  InertiaType=CalculateFromGeometry  BasedOnType=Density  Density=handDensity  DensityUnits=kg/m^3  Mass=0  MassUnits=kg  CenterOfMass=[0, 0, 0]  CenterOfMassUnits=m  MomentsOfInertia=[0, 0, 0]  MomentsOfInertiaUnits=kg*m^2  ProductsOfInertia=[0, 0, 0]  ProductsOfInertiaUnits=kg*m^2  GraphicType=FromGeometry  MarkerShape=Sphere  MarkerSize=10  GraphicVisPropType=SimpleVisualProperties  GraphicDiffuseColor=[0.3, 0.3, 0.3]  GraphicOpacity=1  GraphicSpecularColor=[0.5 0.5 0.5 1.0]  GraphicAmbientColor=[0.15 0.15 0.15 1.0]  GraphicEmissiveColor=[0.0 0.0 0.0 1.0]  GraphicShininess=75  DoExposeReferenceFrame=on  SerializedFrames=<Frames/>
  Lower Arm : sm_lib/Body Elements/File Solid  ExtGeomFileName=sm_humanoid_walker_lower_arm.stp  UnitType=FromFile  ExtGeomFileUnits=m  StepReaderType=HEX  ExportConvexHullGeometry=off  InertiaType=CalculateFromGeometry  BasedOnType=Density  Density=lowerArmDensity  DensityUnits=kg/m^3  Mass=0  MassUnits=kg  CenterOfMass=[0, 0, 0]  CenterOfMassUnits=m  MomentsOfInertia=[0, 0, 0]  MomentsOfInertiaUnits=kg*m^2  ProductsOfInertia=[0, 0, 0]  ProductsOfInertiaUnits=kg*m^2  GraphicType=FromGeometry  MarkerShape=Sphere  MarkerSize=10  GraphicVisPropType=SimpleVisualProperties  GraphicDiffuseColor=[1, 1, 1]  GraphicOpacity=1  GraphicSpecularColor=[0.5 0.5 0.5 1.0]  GraphicAmbientColor=[0.15 0.15 0.15 1.0]  GraphicEmissiveColor=[0.0 0.0 0.0 1.0]  GraphicShininess=75  DoExposeReferenceFrame=on  SerializedFrames=<Frames/>
  Shoulder Frontal Joint : Subsystem
  Shoulder Sagittal Joint : Subsystem
  Shoulder Swivel : sm_lib/Body Elements/File Solid  ExtGeomFileName=sm_humanoid_walker_shoulder_swivel.stp  UnitType=FromFile  ExtGeomFileUnits=m  StepReaderType=HEX  ExportConvexHullGeometry=off  InertiaType=CalculateFromGeometry  BasedOnType=Density  Density=shoulderDensity  DensityUnits=kg/m^3  Mass=0  MassUnits=kg  CenterOfMass=[0, 0, 0]  CenterOfMassUnits=m  MomentsOfInertia=[0, 0, 0]  MomentsOfInertiaUnits=kg*m^2  ProductsOfInertia=[0, 0, 0]  ProductsOfInertiaUnits=kg*m^2  GraphicType=FromGeometry  MarkerShape=Sphere  MarkerSize=10  GraphicVisPropType=SimpleVisualProperties  GraphicDiffuseColor=[0.3, 0.3, 0.3]  GraphicOpacity=1  GraphicSpecularColor=[0.5 0.5 0.5 1.0]  GraphicAmbientColor=[0.15 0.15 0.15 1.0]  GraphicEmissiveColor=[0.0 0.0 0.0 1.0]  GraphicShininess=75  DoExposeReferenceFrame=on  SerializedFrames=<Frames/>
  Upper Arm : sm_lib/Body Elements/File Solid  ExtGeomFileName=sm_humanoid_walker_upper_arm.stp  UnitType=FromFile  ExtGeomFileUnits=m  StepReaderType=HEX  ExportConvexHullGeometry=off  InertiaType=CalculateFromGeometry  BasedOnType=Density  Density=upperArmDensity  DensityUnits=kg/m^3  Mass=0  MassUnits=kg  CenterOfMass=[0, 0, 0]  CenterOfMassUnits=m  MomentsOfInertia=[0, 0, 0]  MomentsOfInertiaUnits=kg*m^2  ProductsOfInertia=[0, 0, 0]  ProductsOfInertiaUnits=kg*m^2  GraphicType=FromGeometry  MarkerShape=Sphere  MarkerSize=10  GraphicVisPropType=SimpleVisualProperties  GraphicDiffuseColor=[1, 1, 1]  GraphicOpacity=1  GraphicSpecularColor=[0.5 0.5 0.5 1.0]  GraphicAmbientColor=[0.15 0.15 0.15 1.0]  GraphicEmissiveColor=[0.0 0.0 0.0 1.0]  GraphicShininess=75  DoExposeReferenceFrame=on  SerializedFrames=<Frames/>
  Wrist Joint : Subsystem
  Left Shoulder : PMIOPort  Side=Left
  connections:
  Upper Arm/RConn1 -- Shoulder Sagittal Joint/RConn1 -- Elbow Joint/LConn1
  Shoulder Frontal Joint/RConn1 -- Shoulder Swivel/RConn1 -- Shoulder Sagittal Joint/LConn1
  Shoulder Frontal Joint/LConn1 -- Left Shoulder/RConn1
  Lower Arm/RConn1 -- Elbow Joint/RConn1 -- Wrist Joint/LConn1
  Wrist Joint/RConn1 -- Hand/RConn1

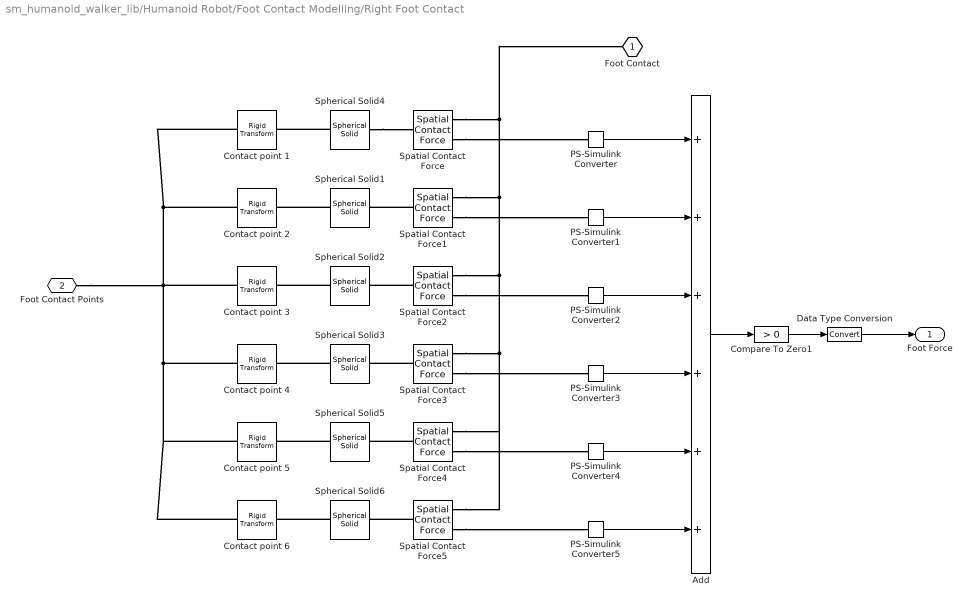
== system sm_humanoid_walker_lib/Humanoid Robot/Foot Contact Modelling/Right Foot Contact ==
  Add : Sum  Inputs=++++++
  Compare To Zero1 : simulink/Logic and Bit Operations/Compare To Zero  relop=>  OutDataTypeStr=boolean  ZeroCross=off
  Contact point 1 : sm_lib/Frames and Transforms/Rigid Transform  RotationMethod=RotationSequence  FollAlignAxisA=+X  BaseAlignAxisA=+Y  FollAlignAxisB=+Y  BaseAlignAxisB=+Z  RotationStandardAxis=+Z  RotationAngle=0.0  RotationAngleUnits=deg  RotationArbitraryAxis=[0 0 1]  RotationSequenceAxes=BaseAxes  RotationSequence=XYZ  RotationSequenceAngles=[0, 0, 0]  RotationSequenceAnglesUnits=rad  RotationMatrix=[1 0 0; 0 1 0; 0 0 1]  Quaternion=[1 0 0 0]  TranslationMethod=Cartesian  TranslationCartesianOffset=[0.035 0.03, -0.026]*3.5*0.9  TranslationCartesianOffsetUnits=m  TranslationStandardAxis=+Z  TranslationStandardOffset=0  TranslationStandardOffsetUnits=m  TranslationROffset=0  TranslationROffsetUnits=m  TranslationThetaOffset=0  TranslationThetaOffsetUnits=deg  TranslationZOffset=0  TranslationZOffsetUnits=m
  Contact point 2 : sm_lib/Frames and Transforms/Rigid Transform  RotationMethod=RotationSequence  FollAlignAxisA=+X  BaseAlignAxisA=+Y  FollAlignAxisB=+Y  BaseAlignAxisB=+Z  RotationStandardAxis=+Z  RotationAngle=0.0  RotationAngleUnits=deg  RotationArbitraryAxis=[0 0 1]  RotationSequenceAxes=BaseAxes  RotationSequence=XYZ  RotationSequenceAngles=[0, 0, 0]  RotationSequenceAnglesUnits=rad  RotationMatrix=[1 0 0; 0 1 0; 0 0 1]  Quaternion=[1 0 0 0]  TranslationMethod=Cartesian  TranslationCartesianOffset=[-0.035, 0.03, -0.026]*3.5*0.9  TranslationCartesianOffsetUnits=m  TranslationStandardAxis=+Z  TranslationStandardOffset=0  TranslationStandardOffsetUnits=m  TranslationROffset=0  TranslationROffsetUnits=m  TranslationThetaOffset=0  TranslationThetaOffsetUnits=deg  TranslationZOffset=0  TranslationZOffsetUnits=m
  Contact point 3 : sm_lib/Frames and Transforms/Rigid Transform  RotationMethod=RotationSequence  FollAlignAxisA=+X  BaseAlignAxisA=+Y  FollAlignAxisB=+Y  BaseAlignAxisB=+Z  RotationStandardAxis=+Z  RotationAngle=0.0  RotationAngleUnits=deg  RotationArbitraryAxis=[0 0 1]  RotationSequenceAxes=BaseAxes  RotationSequence=XYZ  RotationSequenceAngles=[0, 0, 0]  RotationSequenceAnglesUnits=rad  RotationMatrix=[1 0 0; 0 1 0; 0 0 1]  Quaternion=[1 0 0 0]  TranslationMethod=Cartesian  TranslationCartesianOffset=[-0.035, -0.065, -0.026]*3.5*0.9  TranslationCartesianOffsetUnits=m  TranslationStandardAxis=+Z  TranslationStandardOffset=0  TranslationStandardOffsetUnits=m  TranslationROffset=0  TranslationROffsetUnits=m  TranslationThetaOffset=0  TranslationThetaOffsetUnits=deg  TranslationZOffset=0  TranslationZOffsetUnits=m
  Contact point 4 : sm_lib/Frames and Transforms/Rigid Transform  RotationMethod=RotationSequence  FollAlignAxisA=+X  BaseAlignAxisA=+Y  FollAlignAxisB=+Y  BaseAlignAxisB=+Z  RotationStandardAxis=+Z  RotationAngle=0.0  RotationAngleUnits=deg  RotationArbitraryAxis=[0 0 1]  RotationSequenceAxes=BaseAxes  RotationSequence=XYZ  RotationSequenceAngles=[0, 0, 0]  RotationSequenceAnglesUnits=rad  RotationMatrix=[1 0 0; 0 1 0; 0 0 1]  Quaternion=[1 0 0 0]  TranslationMethod=Cartesian  TranslationCartesianOffset=[0.035, -0.065, -0.026]*3.5*0.9  TranslationCartesianOffsetUnits=m  TranslationStandardAxis=+Z  TranslationStandardOffset=0  TranslationStandardOffsetUnits=m  TranslationROffset=0  TranslationROffsetUnits=m  TranslationThetaOffset=0  TranslationThetaOffsetUnits=deg  TranslationZOffset=0  TranslationZOffsetUnits=m
  Contact point 5 : sm_lib/Frames and Transforms/Rigid Transform  RotationMethod=RotationSequence  FollAlignAxisA=+X  BaseAlignAxisA=+Y  FollAlignAxisB=+Y  BaseAlignAxisB=+Z  RotationStandardAxis=+Z  RotationAngle=0.0  RotationAngleUnits=deg  RotationArbitraryAxis=[0 0 1]  RotationSequenceAxes=BaseAxes  RotationSequence=XYZ  RotationSequenceAngles=[0, 0, 0]  RotationSequenceAnglesUnits=rad  RotationMatrix=[1 0 0; 0 1 0; 0 0 1]  Quaternion=[1 0 0 0]  TranslationMethod=Cartesian  TranslationCartesianOffset=[0.035, -0.085, -0.02]*3.5*0.9  TranslationCartesianOffsetUnits=m  TranslationStandardAxis=+Z  TranslationStandardOffset=0  TranslationStandardOffsetUnits=m  TranslationROffset=0  TranslationROffsetUnits=m  TranslationThetaOffset=0  TranslationThetaOffsetUnits=deg  TranslationZOffset=0  TranslationZOffsetUnits=m
  Contact point 6 : sm_lib/Frames and Transforms/Rigid Transform  RotationMethod=RotationSequence  FollAlignAxisA=+X  BaseAlignAxisA=+Y  FollAlignAxisB=+Y  BaseAlignAxisB=+Z  RotationStandardAxis=+Z  RotationAngle=0.0  RotationAngleUnits=deg  RotationArbitraryAxis=[0 0 1]  RotationSequenceAxes=BaseAxes  RotationSequence=XYZ  RotationSequenceAngles=[0, 0, 0]  RotationSequenceAnglesUnits=rad  RotationMatrix=[1 0 0; 0 1 0; 0 0 1]  Quaternion=[1 0 0 0]  TranslationMethod=Cartesian  TranslationCartesianOffset=[-0.035, -0.085, -0.02]*3.5*0.9  TranslationCartesianOffsetUnits=m  TranslationStandardAxis=+Z  TranslationStandardOffset=0  TranslationStandardOffsetUnits=m  TranslationROffset=0  TranslationROffsetUnits=m  TranslationThetaOffset=0  TranslationThetaOffsetUnits=deg  TranslationZOffset=0  TranslationZOffsetUnits=m
  Data Type Conversion : DataTypeConversion  SaturateOnIntegerOverflow=off  RndMeth=Floor
  PS-Simulink Converter{,1..5} (6 alike) : nesl_utility/PS-Simulink Converter  PhysicalDomain=network_engine_domain  SubClassName=ps_output  LeftPortType=input  RightPortType=output  PseudoPeriodic=off  Frequencies=[]  VectorFormat=1-D array  Unit=inherit  AffineConversion=off
  Spatial Contact Force{,1..5} (6 alike) : sm_lib/Forces and Torques/Spatial Contact Force  SenseSeparationDistance=off  NormalForceType=SmoothSpringDamper  NormalStiffness=contactStiffness  NormalStiffnessUnits=N/m  NormalDamping=contactDamping  NormalDampingUnits=N/(m/s)  NormalTransitionRegionWidth=contactTWidth  NormalTransitionRegionWidthUnits=m  FrictionType=SmoothStickSlip  CoefficientOfStaticFriction=contactStaticFriction  CoefficientOfDynamicFriction=contactDynamicFriction  FrictionalCriticalVelocity=contactCriticalVelocity  FrictionalCriticalVelocityUnits=m/s  SenseContactSignal=off  SensePenetrationDepth=off  SenseNormalVelocity=off  SenseTangentialVelocity=off  SensingForceTorqueDirection=BaseOnFollower  SensingForceTorqueResolutionFrame=ContactFrame  SenseNormalForce=off  SenseNormalForceMagnitude=on  SenseNormalTorque=off  SenseFrictionalForce=off  SenseFrictionalForceMagnitude=off  SenseFrictionalTorque=off  SenseTotalForce=off  SenseTotalTorque=off  SenseContactBaseRotation=off  SenseContactBaseTranslation=off  SenseContactFollowerRotation=off  SenseContactFollowerTranslation=off  ZeroCrossDetectContactStartAndEnd=off
  Spherical Solid{1..6} (6 alike) : sm_lib/Body Elements/Spherical Solid  SphereRadius=contactRadius  SphereRadiusUnits=m  ExportEntireGeometry=on  InertiaType=CalculateFromGeometry  BasedOnType=Density  Density=0  DensityUnits=kg/m^3  Mass=1  MassUnits=kg  CenterOfMass=[0 0 0]  CenterOfMassUnits=m  MomentsOfInertia=[1 1 1]  MomentsOfInertiaUnits=kg*m^2  ProductsOfInertia=[0 0 0]  ProductsOfInertiaUnits=kg*m^2  GraphicType=None  MarkerShape=Sphere  MarkerSize=10  GraphicVisPropType=SimpleVisualProperties  GraphicDiffuseColor=[1.0 0.0 0.0]  GraphicOpacity=1.0  GraphicSpecularColor=[0.5 0.5 0.5 1.0]  GraphicAmbientColor=[0.15 0.15 0.15 1.0]  GraphicEmissiveColor=[0.0 0.0 0.0 1.0]  GraphicShininess=75  DoExposeReferenceFrame=on  SerializedFrames=<Frames/>
  Foot Contact : PMIOPort  Side=Right
  Foot Contact Points : PMIOPort  Port=2  Side=Left
  Foot Force : Outport
  wires:
  PS-Simulink Converter5/1 -> Add/6
  PS-Simulink Converter4/1 -> Add/5
  PS-Simulink Converter3/1 -> Add/4
  PS-Simulink Converter2/1 -> Add/3
  PS-Simulink Converter1/1 -> Add/2
  Data Type Conversion/1 -> Foot Force/1
  Add/1 -> Compare To Zero1/1
  Compare To Zero1/1 -> Data Type Conversion/1
  PS-Simulink Converter/1 -> Add/1
  connections:
  Spatial Contact Force4/RConn2 -- PS-Simulink Converter4/LConn1
  Spatial Contact Force4/LConn1 -- Spherical Solid5/LConn1
  Spatial Contact Force5/RConn2 -- PS-Simulink Converter5/LConn1
  Spatial Contact Force5/LConn1 -- Spherical Solid6/LConn1
  Spherical Solid6/RConn1 -- Contact point 6/RConn1
  Spherical Solid5/RConn1 -- Contact point 5/RConn1
  Spatial Contact Force1/LConn1 -- Spherical Solid1/LConn1
  Spatial Contact Force2/LConn1 -- Spherical Solid2/LConn1
  Spatial Contact Force3/LConn1 -- Spherical Solid3/LConn1
  Spherical Solid4/LConn1 -- Spatial Contact Force/LConn1
  Spherical Solid2/RConn1 -- Contact point 3/RConn1
  Spherical Solid1/RConn1 -- Contact point 2/RConn1
  Spherical Solid4/RConn1 -- Contact point 1/RConn1
  Spatial Contact Force5/RConn1 -- Spatial Contact Force4/RConn1 -- Spatial Contact Force3/RConn1 -- Spatial Contact Force2/RConn1 -- Spatial Contact Force1/RConn1 -- Foot Contact/RConn1 -- Spatial Contact Force/RConn1
  Spherical Solid3/RConn1 -- Contact point 4/RConn1
  Spatial Contact Force2/RConn2 -- PS-Simulink Converter2/LConn1
  Spatial Contact Force/RConn2 -- PS-Simulink Converter/LConn1
  Spatial Contact Force3/RConn2 -- PS-Simulink Converter3/LConn1
  Spatial Contact Force1/RConn2 -- PS-Simulink Converter1/LConn1
  Foot Contact Points/RConn1 -- Contact point 3/LConn1 -- Contact point 4/LConn1 -- Contact point 5/LConn1 -- Contact point 6/LConn1 -- Contact point 2/LConn1 -- Contact point 1/LConn1
